simulink model "sevietta_devel_2017h"  (R2013a)
settings: Solver=VariableStepDiscrete  SolverMode=SingleTasking  StartTime=0.0  StopTime=3276  RelTol=1e-3
undefined symbols (not defined in the file): sfp
libraries: xbsIndex_r4 x2565, casper_library_delays x32, simulink x19, casper_library_misc x17, xps_library x13
(part 24 of 31)

== system sevietta_devel_2017h/pkt/packetizer/pkt_header ==
  note: CHIPS 2.0: Spare byte before first_chan
  note: trigger signal does selection on mux
  rst : Inport
  new_seq : Inport  Port=2
  new_pkt : Inport  Port=3
  roach_id : Inport  Port=4
  gbe_id : Inport  Port=5
  n_chan : Inport  Port=6
  n_subband : Inport  Port=7
  subband_id : Inport  Port=8
  first_chan : Inport  Port=9
  spare : Inport  Port=10
  Concat : xbsIndex_r4/Concat  num_inputs=7  dbl_ovrd=off  block_type=concat
  Delay1 : xbsIndex_r4/Delay  rst=off  infoeditControl=Selection of Reset will increase slice count due to use of real FFs and instead of SRLs  en=off  latency=4  dbl_ovrd=off  reg_retiming=off  block_type=delay
  Delay2 : xbsIndex_r4/Delay  rst=off  infoeditControl=Selection of Reset will increase slice count due to use of real FFs and instead of SRLs  en=off  latency=2  dbl_ovrd=off  reg_retiming=off  block_type=delay
  Delay3 : xbsIndex_r4/Delay  rst=off  infoeditControl=Selection of Reset will increase slice count due to use of real FFs and instead of SRLs  en=off  latency=4  dbl_ovrd=off  reg_retiming=off  block_type=delay
  Gateway Out{1..4,8} (5 alike) : xbsIndex_r4/Gateway Out  inherit_from_input=off  hdl_port=on  timing_constraint=None  locs_specified=off  LOCs={}  UseAsDAC=off  DACChannel='1'  block_type=gatewayout
  Mux : xbsIndex_r4/Mux  inputs=2  en=off  latency=1  precision=Full  arith_type=Unsigned  n_bits=16  bin_pt=14  quantization=Truncate  overflow=Wrap  dbl_ovrd=off  block_type=mux
  Scope2 : Scope  NumInputPorts=5
      settings: ShowLegends=on  TimeRange=50000  YMin=-5~0~-5~0~-5  YMax=5~8e+16~5~10~5  SaveName=ScopeData2  MaxDataPoints=10000
  Slice{,1..4,6} (6 alike) : xbsIndex_r4/Slice  nbits=8  boolean_output=off  mode=Lower Bit Location + Width  bit1=0  base1=MSB of Input  bit0=0  base0=LSB of Input  dbl_ovrd=off  block_type=slice
  Slice5 : xbsIndex_r4/Slice  nbits=16  boolean_output=off  mode=Lower Bit Location + Width  bit1=0  base1=MSB of Input  bit0=0  base0=LSB of Input  dbl_ovrd=off  block_type=slice
  pulse_ext : casper_library_misc/pulse_ext  pulse_len=2
  seq_no : xbsIndex_r4/Counter  cnt_type=Free Running  cnt_to=Inf  operation=Up  start_count=0  cnt_by_val=1  arith_type=Unsigned  n_bits=64  bin_pt=0  load_pin=off  rst=on  en=on  explicit_period=on  period=1  dbl_ovrd=off  use_behavioral_HDL=off  implementation=Fabric  block_type=counter
  hdr_valid : Outport
  hdr_out : Outport  Port=2
  wires:
  Delay2/1 -> pulse_ext/1, Gateway Out1/1, Mux/1
  first_chan/1 -> Slice5/1
  subband_id/1 -> Slice4/1
  spare/1 -> Slice6/1
  Slice4/1 -> Concat/5
  pulse_ext/1 -> Delay1/1
  Mux/1 -> Delay3/1
  gbe_id/1 -> Slice1/1
  new_seq/1 -> seq_no/2
  n_subband/1 -> Slice3/1
  Slice1/1 -> Concat/2
  Slice/1 -> Concat/1
  n_chan/1 -> Slice2/1
  rst/1 -> seq_no/1
  Slice2/1 -> Concat/3
  Slice3/1 -> Concat/4
  seq_no/1 -> Gateway Out2/1, Mux/2
  roach_id/1 -> Slice/1
  new_pkt/1 -> Delay2/1
  Delay1/1 -> Gateway Out4/1, hdr_valid/1
  Delay3/1 -> Gateway Out8/1, hdr_out/1
  Slice6/1 -> Concat/6
  Slice5/1 -> Concat/7
  Gateway Out1/1 -> Scope2/1  "new_pkt"
  Gateway Out2/1 -> Scope2/2  "seq_no"
  Gateway Out3/1 -> Scope2/3  "hdr_data"
  Gateway Out8/1 -> Scope2/4  "output"
  Gateway Out4/1 -> Scope2/5
  Concat/1 -> Mux/3, Gateway Out3/1

== system sevietta_devel_2017h/pkt/packetizer/re_logic ==
  sow : Inport
  n_chanps : Inport  Port=2
  n_subband : Inport  Port=3
  cnt_rst : Inport  Port=4
  start_chan : Inport  Port=5
  Delay4 : xbsIndex_r4/Delay  rst=off  infoeditControl=Selection of Reset will increase slice count due to use of real FFs and instead of SRLs  en=off  latency=5  dbl_ovrd=off  reg_retiming=off  block_type=delay
  Delay5 : xbsIndex_r4/Delay  rst=off  infoeditControl=Selection of Reset will increase slice count due to use of real FFs and instead of SRLs  en=off  latency=5  dbl_ovrd=off  reg_retiming=off  block_type=delay
  Delay6 : xbsIndex_r4/Delay  rst=off  infoeditControl=Selection of Reset will increase slice count due to use of real FFs and instead of SRLs  en=off  latency=5  dbl_ovrd=off  reg_retiming=off  block_type=delay
  Delay7 : xbsIndex_r4/Delay  rst=off  infoeditControl=Selection of Reset will increase slice count due to use of real FFs and instead of SRLs  en=off  latency=1  dbl_ovrd=off  reg_retiming=off  block_type=delay
  compute_pkt_chan1 : Subsystem
  gen_eof1 : Subsystem
  re_logic1 : Subsystem
  new_cycle_out : Outport
  sub_id_out : Outport  Port=2
  sub_re : Outport  Port=3
  sof : Outport  Port=4
  eof : Outport  Port=5
  pkt_chan0 : Outport  Port=6
  wires:
  Delay6/1 -> gen_eof1/3(subband_re)
  compute_pkt_chan1/1(pkt_chan0) -> Delay7/1
  Delay7/1 -> pkt_chan0/1
  sow/1 -> re_logic1/1(sow)
  gen_eof1/5(eof) -> eof/1
  gen_eof1/4(sof) -> sof/1
  gen_eof1/2(subband_id_out) -> sub_id_out/1
  gen_eof1/3(pkt_re) -> sub_re/1
  n_subband/1 -> re_logic1/3(n_subband)
  n_chanps/1 -> compute_pkt_chan1/1(n_chanps), re_logic1/2(n_chanps)
  cnt_rst/1 -> re_logic1/4(rst)
  start_chan/1 -> compute_pkt_chan1/3(start_chan)
  Delay4/1 -> gen_eof1/1(new_cycle)
  Delay5/1 -> gen_eof1/2(subband_id)
  re_logic1/1(new_cycle) -> Delay4/1
  re_logic1/3(subband_re) -> Delay6/1
  re_logic1/2(subband_id) -> compute_pkt_chan1/2(subband_id), Delay5/1
  gen_eof1/1(new_cycle_out) -> new_cycle_out/1

== system sevietta_devel_2017h/pkt/packetizer1/pkt_buffer ==
  note: LATENCY TO MATCH FIFO LATENCY
  re : Inport
  d_in : Inport  Port=2
  we : Inport  Port=3
  new_fft_win : Inport  Port=4
  Constant1 : xbsIndex_r4/Constant  const=0  gui_display_data_type=Fixed-point  arith_type=Unsigned  n_bits=64  bin_pt=0  preci_type=Single  exp_width=8  frac_width=24  explicit_period=on  period=1  equ=P=C  opselect=C  inp2=PCIN>>17  opr=+  inp1=P  carry=CIN  dbl_ovrd=off  block_type=constant
  Constant2 : xbsIndex_r4/Constant  const=0  gui_display_data_type=Boolean  arith_type=Boolean  n_bits=64  bin_pt=0  preci_type=Single  exp_width=8  frac_width=24  explicit_period=on  period=1  equ=P=C  opselect=C  inp2=PCIN>>17  opr=+  inp1=P  carry=CIN  dbl_ovrd=off  block_type=constant
  Delay1 : xbsIndex_r4/Delay  rst=off  infoeditControl=Selection of Reset will increase slice count due to use of real FFs and instead of SRLs  en=off  latency=5  dbl_ovrd=off  reg_retiming=off  block_type=delay
  Delay2 : xbsIndex_r4/Delay  rst=off  infoeditControl=Selection of Reset will increase slice count due to use of real FFs and instead of SRLs  en=off  latency=5  dbl_ovrd=off  reg_retiming=off  block_type=delay
  Delay5 : xbsIndex_r4/Delay  rst=off  infoeditControl=Selection of Reset will increase slice count due to use of real FFs and instead of SRLs  en=off  latency=3  dbl_ovrd=off  reg_retiming=off  block_type=delay
  Gateway Out{1..5,7..9,18..20} (11 alike) : xbsIndex_r4/Gateway Out  inherit_from_input=off  hdl_port=on  timing_constraint=None  locs_specified=off  LOCs={}  UseAsDAC=off  DACChannel='1'  block_type=gatewayout
  Scope1 : Scope  NumInputPorts=2
      settings: ShowLegends=on  YMin=-0.1~-0.1  YMax=1.1~1.1  MaxDataPoints=10000
  Scope3 : Scope  NumInputPorts=3
      settings: ShowLegends=on  YMin=-0.1~-0.1~-0.1  YMax=1.1~1.1~1.1  SaveName=ScopeData3  MaxDataPoints=10000
  Scope5 : Scope  NumInputPorts=6
      settings: ShowLegends=on  YMin=-5~-5~-0.1~-5~-5~-0.1  YMax=5~5~1.1~5~5~1.1  MaxDataPoints=10000
  dual_prt_ram : xbsIndex_r4/Dual Port RAM  depth=4096  initVector=sin(pi*(0:15)/16)  distributed_mem=Block RAM  init_a=0  init_b=0  rst_a=off  rst_b=off  en_a=off  en_b=off  latency=3  write_mode_A=Read After Write  write_mode_B=Read After Write  dbl_ovrd=off  optimize=Area  block_type=dpram
  re_addr : xbsIndex_r4/Counter  cnt_type=Free Running  cnt_to=Inf  operation=Up  start_count=0  cnt_by_val=1  arith_type=Unsigned  n_bits=12  bin_pt=0  load_pin=off  rst=on  en=on  explicit_period=on  period=1  dbl_ovrd=off  use_behavioral_HDL=off  implementation=Fabric  block_type=counter
  wr_addr : xbsIndex_r4/Counter  cnt_type=Free Running  cnt_to=Inf  operation=Up  start_count=0  cnt_by_val=1  arith_type=Unsigned  n_bits=10  bin_pt=0  load_pin=off  rst=on  en=on  explicit_period=on  period=1  dbl_ovrd=off  use_behavioral_HDL=off  implementation=Fabric  block_type=counter
  d_valid : Outport
  d_out : Outport  Port=2
  wires:
  Delay2/1 -> d_out/1, Gateway Out5/1
  Delay1/1 -> d_valid/1, Gateway Out4/1
  Constant2/1 -> dual_prt_ram/3, Gateway Out19/1
  re/1 -> Gateway Out9/1, re_addr/2, Delay5/1
  Gateway Out5/1 -> Scope1/2
  Gateway Out4/1 -> Scope1/1
  dual_prt_ram/1 -> Delay2/1
  d_in/1 -> Gateway Out1/1, dual_prt_ram/5
  Constant1/1 -> dual_prt_ram/2, Gateway Out18/1
  Gateway Out3/1 -> Scope5/4  "addr_b"
  Gateway Out1/1 -> Scope5/5  "data_b"
  Gateway Out2/1 -> Scope5/6  "we_b"
  [wr_en] -> dual_prt_ram/6, Gateway Out2/1
  [wr_addr] -> dual_prt_ram/4, Gateway Out3/1
  [re_addr] -> dual_prt_ram/1, Gateway Out20/1
  Gateway Out8/1 -> Scope3/3  "fftwin"
  Gateway Out7/1 -> Scope3/2  "ween"
  Gateway Out9/1 -> Scope3/1  "reen"
  [new_fft_win] -> re_addr/1
  [new_fft_win] -> wr_addr/1
  Gateway Out19/1 -> Scope5/3  "we_a"
  Gateway Out18/1 -> Scope5/2  "data_a"
  Gateway Out20/1 -> Scope5/1  "addr_a"
  wr_addr/1 -> [wr_addr]
  re_addr/1 -> [re_addr]
  new_fft_win/1 -> Gateway Out8/1, [new_fft_win]
  we/1 -> Gateway Out7/1, wr_addr/2, [wr_en]
  Delay5/1 -> Delay1/1

== system sevietta_devel_2017h/pkt/packetizer1/pkt_header ==
  note: trigger signal does selection on mux
  note: CHIPS 2.0: Spare byte before first_chan
  rst : Inport
  new_seq : Inport  Port=2
  new_pkt : Inport  Port=3
  roach_id : Inport  Port=4
  gbe_id : Inport  Port=5
  n_chan : Inport  Port=6
  n_subband : Inport  Port=7
  subband_id : Inport  Port=8
  first_chan : Inport  Port=9
  spare : Inport  Port=10
  Concat : xbsIndex_r4/Concat  num_inputs=7  dbl_ovrd=off  block_type=concat
  Delay1 : xbsIndex_r4/Delay  rst=off  infoeditControl=Selection of Reset will increase slice count due to use of real FFs and instead of SRLs  en=off  latency=4  dbl_ovrd=off  reg_retiming=off  block_type=delay
  Delay2 : xbsIndex_r4/Delay  rst=off  infoeditControl=Selection of Reset will increase slice count due to use of real FFs and instead of SRLs  en=off  latency=2  dbl_ovrd=off  reg_retiming=off  block_type=delay
  Delay3 : xbsIndex_r4/Delay  rst=off  infoeditControl=Selection of Reset will increase slice count due to use of real FFs and instead of SRLs  en=off  latency=4  dbl_ovrd=off  reg_retiming=off  block_type=delay
  Gateway Out{1..4,8} (5 alike) : xbsIndex_r4/Gateway Out  inherit_from_input=off  hdl_port=on  timing_constraint=None  locs_specified=off  LOCs={}  UseAsDAC=off  DACChannel='1'  block_type=gatewayout
  Mux : xbsIndex_r4/Mux  inputs=2  en=off  latency=1  precision=Full  arith_type=Unsigned  n_bits=16  bin_pt=14  quantization=Truncate  overflow=Wrap  dbl_ovrd=off  block_type=mux
  Scope2 : Scope  NumInputPorts=5
      settings: ShowLegends=on  TimeRange=50000  YMin=-5~0~-5~0~-5  YMax=5~8e+16~5~10~5  SaveName=ScopeData2  MaxDataPoints=10000
  Slice{,1..4,6} (6 alike) : xbsIndex_r4/Slice  nbits=8  boolean_output=off  mode=Lower Bit Location + Width  bit1=0  base1=MSB of Input  bit0=0  base0=LSB of Input  dbl_ovrd=off  block_type=slice
  Slice5 : xbsIndex_r4/Slice  nbits=16  boolean_output=off  mode=Lower Bit Location + Width  bit1=0  base1=MSB of Input  bit0=0  base0=LSB of Input  dbl_ovrd=off  block_type=slice
  pulse_ext : casper_library_misc/pulse_ext  pulse_len=2
  seq_no : xbsIndex_r4/Counter  cnt_type=Free Running  cnt_to=Inf  operation=Up  start_count=0  cnt_by_val=1  arith_type=Unsigned  n_bits=64  bin_pt=0  load_pin=off  rst=on  en=on  explicit_period=on  period=1  dbl_ovrd=off  use_behavioral_HDL=off  implementation=Fabric  block_type=counter
  hdr_valid : Outport
  hdr_out : Outport  Port=2
  wires:
  Concat/1 -> Gateway Out3/1, Mux/3
  Gateway Out4/1 -> Scope2/5
  Gateway Out8/1 -> Scope2/4  "output"
  Gateway Out3/1 -> Scope2/3  "hdr_data"
  Gateway Out2/1 -> Scope2/2  "seq_no"
  Gateway Out1/1 -> Scope2/1  "new_pkt"
  Slice5/1 -> Concat/7
  Slice6/1 -> Concat/6
  Delay3/1 -> hdr_out/1, Gateway Out8/1
  Delay1/1 -> hdr_valid/1, Gateway Out4/1
  new_pkt/1 -> Delay2/1
  roach_id/1 -> Slice/1
  seq_no/1 -> Mux/2, Gateway Out2/1
  Slice3/1 -> Concat/4
  Slice2/1 -> Concat/3
  rst/1 -> seq_no/1
  n_chan/1 -> Slice2/1
  Slice/1 -> Concat/1
  Slice1/1 -> Concat/2
  n_subband/1 -> Slice3/1
  new_seq/1 -> seq_no/2
  gbe_id/1 -> Slice1/1
  Mux/1 -> Delay3/1
  pulse_ext/1 -> Delay1/1
  Slice4/1 -> Concat/5
  spare/1 -> Slice6/1
  subband_id/1 -> Slice4/1
  first_chan/1 -> Slice5/1
  Delay2/1 -> Mux/1, Gateway Out1/1, pulse_ext/1

== system sevietta_devel_2017h/pkt/packetizer1/re_logic ==
  sow : Inport
  n_chanps : Inport  Port=2
  n_subband : Inport  Port=3
  cnt_rst : Inport  Port=4
  start_chan : Inport  Port=5
  Delay4 : xbsIndex_r4/Delay  rst=off  infoeditControl=Selection of Reset will increase slice count due to use of real FFs and instead of SRLs  en=off  latency=5  dbl_ovrd=off  reg_retiming=off  block_type=delay
  Delay5 : xbsIndex_r4/Delay  rst=off  infoeditControl=Selection of Reset will increase slice count due to use of real FFs and instead of SRLs  en=off  latency=5  dbl_ovrd=off  reg_retiming=off  block_type=delay
  Delay6 : xbsIndex_r4/Delay  rst=off  infoeditControl=Selection of Reset will increase slice count due to use of real FFs and instead of SRLs  en=off  latency=5  dbl_ovrd=off  reg_retiming=off  block_type=delay
  Delay7 : xbsIndex_r4/Delay  rst=off  infoeditControl=Selection of Reset will increase slice count due to use of real FFs and instead of SRLs  en=off  latency=1  dbl_ovrd=off  reg_retiming=off  block_type=delay
  compute_pkt_chan1 : Subsystem
  gen_eof1 : Subsystem
  re_logic1 : Subsystem
  new_cycle_out : Outport
  sub_id_out : Outport  Port=2
  sub_re : Outport  Port=3
  sof : Outport  Port=4
  eof : Outport  Port=5
  pkt_chan0 : Outport  Port=6
  wires:
  gen_eof1/1(new_cycle_out) -> new_cycle_out/1
  re_logic1/2(subband_id) -> Delay5/1, compute_pkt_chan1/2(subband_id)
  re_logic1/3(subband_re) -> Delay6/1
  re_logic1/1(new_cycle) -> Delay4/1
  Delay5/1 -> gen_eof1/2(subband_id)
  Delay4/1 -> gen_eof1/1(new_cycle)
  start_chan/1 -> compute_pkt_chan1/3(start_chan)
  cnt_rst/1 -> re_logic1/4(rst)
  n_chanps/1 -> re_logic1/2(n_chanps), compute_pkt_chan1/1(n_chanps)
  n_subband/1 -> re_logic1/3(n_subband)
  gen_eof1/3(pkt_re) -> sub_re/1
  gen_eof1/2(subband_id_out) -> sub_id_out/1
  gen_eof1/4(sof) -> sof/1
  gen_eof1/5(eof) -> eof/1
  sow/1 -> re_logic1/1(sow)
  Delay7/1 -> pkt_chan0/1
  compute_pkt_chan1/1(pkt_chan0) -> Delay7/1
  Delay6/1 -> gen_eof1/3(subband_re)

== system sevietta_devel_2017h/pkt/packetizer2/pkt_buffer ==
  note: LATENCY TO MATCH FIFO LATENCY
  re : Inport
  d_in : Inport  Port=2
  we : Inport  Port=3
  new_fft_win : Inport  Port=4
  Constant1 : xbsIndex_r4/Constant  const=0  gui_display_data_type=Fixed-point  arith_type=Unsigned  n_bits=64  bin_pt=0  preci_type=Single  exp_width=8  frac_width=24  explicit_period=on  period=1  equ=P=C  opselect=C  inp2=PCIN>>17  opr=+  inp1=P  carry=CIN  dbl_ovrd=off  block_type=constant
  Constant2 : xbsIndex_r4/Constant  const=0  gui_display_data_type=Boolean  arith_type=Boolean  n_bits=64  bin_pt=0  preci_type=Single  exp_width=8  frac_width=24  explicit_period=on  period=1  equ=P=C  opselect=C  inp2=PCIN>>17  opr=+  inp1=P  carry=CIN  dbl_ovrd=off  block_type=constant
  Delay1 : xbsIndex_r4/Delay  rst=off  infoeditControl=Selection of Reset will increase slice count due to use of real FFs and instead of SRLs  en=off  latency=5  dbl_ovrd=off  reg_retiming=off  block_type=delay
  Delay2 : xbsIndex_r4/Delay  rst=off  infoeditControl=Selection of Reset will increase slice count due to use of real FFs and instead of SRLs  en=off  latency=5  dbl_ovrd=off  reg_retiming=off  block_type=delay
  Delay5 : xbsIndex_r4/Delay  rst=off  infoeditControl=Selection of Reset will increase slice count due to use of real FFs and instead of SRLs  en=off  latency=3  dbl_ovrd=off  reg_retiming=off  block_type=delay
  Gateway Out{1..5,7..9,18..20} (11 alike) : xbsIndex_r4/Gateway Out  inherit_from_input=off  hdl_port=on  timing_constraint=None  locs_specified=off  LOCs={}  UseAsDAC=off  DACChannel='1'  block_type=gatewayout
  Scope1 : Scope  NumInputPorts=2
      settings: ShowLegends=on  YMin=-0.1~-0.1  YMax=1.1~1.1  MaxDataPoints=10000
  Scope3 : Scope  NumInputPorts=3
      settings: ShowLegends=on  YMin=-0.1~-0.1~-0.1  YMax=1.1~1.1~1.1  SaveName=ScopeData3  MaxDataPoints=10000
  Scope5 : Scope  NumInputPorts=6
      settings: ShowLegends=on  YMin=-5~-5~-0.1~-5~-5~-0.1  YMax=5~5~1.1~5~5~1.1  MaxDataPoints=10000
  dual_prt_ram : xbsIndex_r4/Dual Port RAM  depth=4096  initVector=sin(pi*(0:15)/16)  distributed_mem=Block RAM  init_a=0  init_b=0  rst_a=off  rst_b=off  en_a=off  en_b=off  latency=3  write_mode_A=Read After Write  write_mode_B=Read After Write  dbl_ovrd=off  optimize=Area  block_type=dpram
  re_addr : xbsIndex_r4/Counter  cnt_type=Free Running  cnt_to=Inf  operation=Up  start_count=0  cnt_by_val=1  arith_type=Unsigned  n_bits=12  bin_pt=0  load_pin=off  rst=on  en=on  explicit_period=on  period=1  dbl_ovrd=off  use_behavioral_HDL=off  implementation=Fabric  block_type=counter
  wr_addr : xbsIndex_r4/Counter  cnt_type=Free Running  cnt_to=Inf  operation=Up  start_count=0  cnt_by_val=1  arith_type=Unsigned  n_bits=10  bin_pt=0  load_pin=off  rst=on  en=on  explicit_period=on  period=1  dbl_ovrd=off  use_behavioral_HDL=off  implementation=Fabric  block_type=counter
  d_valid : Outport
  d_out : Outport  Port=2
  wires:
  Delay5/1 -> Delay1/1
  we/1 -> [wr_en], wr_addr/2, Gateway Out7/1
  new_fft_win/1 -> [new_fft_win], Gateway Out8/1
  re_addr/1 -> [re_addr]
  wr_addr/1 -> [wr_addr]
  Gateway Out20/1 -> Scope5/1  "addr_a"
  Gateway Out18/1 -> Scope5/2  "data_a"
  Gateway Out19/1 -> Scope5/3  "we_a"
  [new_fft_win] -> wr_addr/1
  [new_fft_win] -> re_addr/1
  Gateway Out9/1 -> Scope3/1  "reen"
  Gateway Out7/1 -> Scope3/2  "ween"
  Gateway Out8/1 -> Scope3/3  "fftwin"
  [re_addr] -> Gateway Out20/1, dual_prt_ram/1
  [wr_addr] -> Gateway Out3/1, dual_prt_ram/4
  [wr_en] -> Gateway Out2/1, dual_prt_ram/6
  Gateway Out2/1 -> Scope5/6  "we_b"
  Gateway Out1/1 -> Scope5/5  "data_b"
  Gateway Out3/1 -> Scope5/4  "addr_b"
  Constant1/1 -> Gateway Out18/1, dual_prt_ram/2
  d_in/1 -> dual_prt_ram/5, Gateway Out1/1
  dual_prt_ram/1 -> Delay2/1
  Gateway Out4/1 -> Scope1/1
  Gateway Out5/1 -> Scope1/2
  re/1 -> Delay5/1, re_addr/2, Gateway Out9/1
  Constant2/1 -> Gateway Out19/1, dual_prt_ram/3
  Delay1/1 -> Gateway Out4/1, d_valid/1
  Delay2/1 -> Gateway Out5/1, d_out/1

== system sevietta_devel_2017h/pkt/packetizer2/pkt_header ==
  note: CHIPS 2.0: Spare byte before first_chan
  note: trigger signal does selection on mux
  rst : Inport
  new_seq : Inport  Port=2
  new_pkt : Inport  Port=3
  roach_id : Inport  Port=4
  gbe_id : Inport  Port=5
  n_chan : Inport  Port=6
  n_subband : Inport  Port=7
  subband_id : Inport  Port=8
  first_chan : Inport  Port=9
  spare : Inport  Port=10
  Concat : xbsIndex_r4/Concat  num_inputs=7  dbl_ovrd=off  block_type=concat
  Delay1 : xbsIndex_r4/Delay  rst=off  infoeditControl=Selection of Reset will increase slice count due to use of real FFs and instead of SRLs  en=off  latency=4  dbl_ovrd=off  reg_retiming=off  block_type=delay
  Delay2 : xbsIndex_r4/Delay  rst=off  infoeditControl=Selection of Reset will increase slice count due to use of real FFs and instead of SRLs  en=off  latency=2  dbl_ovrd=off  reg_retiming=off  block_type=delay
  Delay3 : xbsIndex_r4/Delay  rst=off  infoeditControl=Selection of Reset will increase slice count due to use of real FFs and instead of SRLs  en=off  latency=4  dbl_ovrd=off  reg_retiming=off  block_type=delay
  Gateway Out{1..4,8} (5 alike) : xbsIndex_r4/Gateway Out  inherit_from_input=off  hdl_port=on  timing_constraint=None  locs_specified=off  LOCs={}  UseAsDAC=off  DACChannel='1'  block_type=gatewayout
  Mux : xbsIndex_r4/Mux  inputs=2  en=off  latency=1  precision=Full  arith_type=Unsigned  n_bits=16  bin_pt=14  quantization=Truncate  overflow=Wrap  dbl_ovrd=off  block_type=mux
  Scope2 : Scope  NumInputPorts=5
      settings: ShowLegends=on  TimeRange=50000  YMin=-5~0~-5~0~-5  YMax=5~8e+16~5~10~5  SaveName=ScopeData2  MaxDataPoints=10000
  Slice{,1..4,6} (6 alike) : xbsIndex_r4/Slice  nbits=8  boolean_output=off  mode=Lower Bit Location + Width  bit1=0  base1=MSB of Input  bit0=0  base0=LSB of Input  dbl_ovrd=off  block_type=slice
  Slice5 : xbsIndex_r4/Slice  nbits=16  boolean_output=off  mode=Lower Bit Location + Width  bit1=0  base1=MSB of Input  bit0=0  base0=LSB of Input  dbl_ovrd=off  block_type=slice
  pulse_ext : casper_library_misc/pulse_ext  pulse_len=2
  seq_no : xbsIndex_r4/Counter  cnt_type=Free Running  cnt_to=Inf  operation=Up  start_count=0  cnt_by_val=1  arith_type=Unsigned  n_bits=64  bin_pt=0  load_pin=off  rst=on  en=on  explicit_period=on  period=1  dbl_ovrd=off  use_behavioral_HDL=off  implementation=Fabric  block_type=counter
  hdr_valid : Outport
  hdr_out : Outport  Port=2
  wires:
  Delay2/1 -> pulse_ext/1, Gateway Out1/1, Mux/1
  first_chan/1 -> Slice5/1
  subband_id/1 -> Slice4/1
  spare/1 -> Slice6/1
  Slice4/1 -> Concat/5
  pulse_ext/1 -> Delay1/1
  Mux/1 -> Delay3/1
  gbe_id/1 -> Slice1/1
  new_seq/1 -> seq_no/2
  n_subband/1 -> Slice3/1
  Slice1/1 -> Concat/2
  Slice/1 -> Concat/1
  n_chan/1 -> Slice2/1
  rst/1 -> seq_no/1
  Slice2/1 -> Concat/3
  Slice3/1 -> Concat/4
  seq_no/1 -> Gateway Out2/1, Mux/2
  roach_id/1 -> Slice/1
  new_pkt/1 -> Delay2/1
  Delay1/1 -> Gateway Out4/1, hdr_valid/1
  Delay3/1 -> Gateway Out8/1, hdr_out/1
  Slice6/1 -> Concat/6
  Slice5/1 -> Concat/7
  Gateway Out1/1 -> Scope2/1  "new_pkt"
  Gateway Out2/1 -> Scope2/2  "seq_no"
  Gateway Out3/1 -> Scope2/3  "hdr_data"
  Gateway Out8/1 -> Scope2/4  "output"
  Gateway Out4/1 -> Scope2/5
  Concat/1 -> Mux/3, Gateway Out3/1

== system sevietta_devel_2017h/pkt/packetizer2/re_logic ==
  sow : Inport
  n_chanps : Inport  Port=2
  n_subband : Inport  Port=3
  cnt_rst : Inport  Port=4
  start_chan : Inport  Port=5
  Delay4 : xbsIndex_r4/Delay  rst=off  infoeditControl=Selection of Reset will increase slice count due to use of real FFs and instead of SRLs  en=off  latency=5  dbl_ovrd=off  reg_retiming=off  block_type=delay
  Delay5 : xbsIndex_r4/Delay  rst=off  infoeditControl=Selection of Reset will increase slice count due to use of real FFs and instead of SRLs  en=off  latency=5  dbl_ovrd=off  reg_retiming=off  block_type=delay
  Delay6 : xbsIndex_r4/Delay  rst=off  infoeditControl=Selection of Reset will increase slice count due to use of real FFs and instead of SRLs  en=off  latency=5  dbl_ovrd=off  reg_retiming=off  block_type=delay
  Delay7 : xbsIndex_r4/Delay  rst=off  infoeditControl=Selection of Reset will increase slice count due to use of real FFs and instead of SRLs  en=off  latency=1  dbl_ovrd=off  reg_retiming=off  block_type=delay
  compute_pkt_chan1 : Subsystem
  gen_eof1 : Subsystem
  re_logic1 : Subsystem
  new_cycle_out : Outport
  sub_id_out : Outport  Port=2
  sub_re : Outport  Port=3
  sof : Outport  Port=4
  eof : Outport  Port=5
  pkt_chan0 : Outport  Port=6
  wires:
  Delay6/1 -> gen_eof1/3(subband_re)
  compute_pkt_chan1/1(pkt_chan0) -> Delay7/1
  Delay7/1 -> pkt_chan0/1
  sow/1 -> re_logic1/1(sow)
  gen_eof1/5(eof) -> eof/1
  gen_eof1/4(sof) -> sof/1
  gen_eof1/2(subband_id_out) -> sub_id_out/1
  gen_eof1/3(pkt_re) -> sub_re/1
  n_subband/1 -> re_logic1/3(n_subband)
  n_chanps/1 -> compute_pkt_chan1/1(n_chanps), re_logic1/2(n_chanps)
  cnt_rst/1 -> re_logic1/4(rst)
  start_chan/1 -> compute_pkt_chan1/3(start_chan)
  Delay4/1 -> gen_eof1/1(new_cycle)
  Delay5/1 -> gen_eof1/2(subband_id)
  re_logic1/1(new_cycle) -> Delay4/1
  re_logic1/3(subband_re) -> Delay6/1
  re_logic1/2(subband_id) -> compute_pkt_chan1/2(subband_id), Delay5/1
  gen_eof1/1(new_cycle_out) -> new_cycle_out/1

== system sevietta_devel_2017h/pkt/packetizer3/pkt_buffer ==
  note: LATENCY TO MATCH FIFO LATENCY
  re : Inport
  d_in : Inport  Port=2
  we : Inport  Port=3
  new_fft_win : Inport  Port=4
  Constant1 : xbsIndex_r4/Constant  const=0  gui_display_data_type=Fixed-point  arith_type=Unsigned  n_bits=64  bin_pt=0  preci_type=Single  exp_width=8  frac_width=24  explicit_period=on  period=1  equ=P=C  opselect=C  inp2=PCIN>>17  opr=+  inp1=P  carry=CIN  dbl_ovrd=off  block_type=constant
  Constant2 : xbsIndex_r4/Constant  const=0  gui_display_data_type=Boolean  arith_type=Boolean  n_bits=64  bin_pt=0  preci_type=Single  exp_width=8  frac_width=24  explicit_period=on  period=1  equ=P=C  opselect=C  inp2=PCIN>>17  opr=+  inp1=P  carry=CIN  dbl_ovrd=off  block_type=constant
  Delay1 : xbsIndex_r4/Delay  rst=off  infoeditControl=Selection of Reset will increase slice count due to use of real FFs and instead of SRLs  en=off  latency=5  dbl_ovrd=off  reg_retiming=off  block_type=delay
  Delay2 : xbsIndex_r4/Delay  rst=off  infoeditControl=Selection of Reset will increase slice count due to use of real FFs and instead of SRLs  en=off  latency=5  dbl_ovrd=off  reg_retiming=off  block_type=delay
  Delay5 : xbsIndex_r4/Delay  rst=off  infoeditControl=Selection of Reset will increase slice count due to use of real FFs and instead of SRLs  en=off  latency=3  dbl_ovrd=off  reg_retiming=off  block_type=delay
  Gateway Out{1..5,7..9,18..20} (11 alike) : xbsIndex_r4/Gateway Out  inherit_from_input=off  hdl_port=on  timing_constraint=None  locs_specified=off  LOCs={}  UseAsDAC=off  DACChannel='1'  block_type=gatewayout
  Scope1 : Scope  NumInputPorts=2
      settings: ShowLegends=on  YMin=-0.1~-0.1  YMax=1.1~1.1  MaxDataPoints=10000
  Scope3 : Scope  NumInputPorts=3
      settings: ShowLegends=on  YMin=-0.1~-0.1~-0.1  YMax=1.1~1.1~1.1  SaveName=ScopeData3  MaxDataPoints=10000
  Scope5 : Scope  NumInputPorts=6
      settings: ShowLegends=on  YMin=-5~-5~-0.1~-5~-5~-0.1  YMax=5~5~1.1~5~5~1.1  MaxDataPoints=10000
  dual_prt_ram : xbsIndex_r4/Dual Port RAM  depth=4096  initVector=sin(pi*(0:15)/16)  distributed_mem=Block RAM  init_a=0  init_b=0  rst_a=off  rst_b=off  en_a=off  en_b=off  latency=3  write_mode_A=Read After Write  write_mode_B=Read After Write  dbl_ovrd=off  optimize=Area  block_type=dpram
  re_addr : xbsIndex_r4/Counter  cnt_type=Free Running  cnt_to=Inf  operation=Up  start_count=0  cnt_by_val=1  arith_type=Unsigned  n_bits=12  bin_pt=0  load_pin=off  rst=on  en=on  explicit_period=on  period=1  dbl_ovrd=off  use_behavioral_HDL=off  implementation=Fabric  block_type=counter
  wr_addr : xbsIndex_r4/Counter  cnt_type=Free Running  cnt_to=Inf  operation=Up  start_count=0  cnt_by_val=1  arith_type=Unsigned  n_bits=10  bin_pt=0  load_pin=off  rst=on  en=on  explicit_period=on  period=1  dbl_ovrd=off  use_behavioral_HDL=off  implementation=Fabric  block_type=counter
  d_valid : Outport
  d_out : Outport  Port=2
  wires:
  Delay2/1 -> d_out/1, Gateway Out5/1
  Delay1/1 -> d_valid/1, Gateway Out4/1
  Constant2/1 -> dual_prt_ram/3, Gateway Out19/1
  re/1 -> Gateway Out9/1, re_addr/2, Delay5/1
  Gateway Out5/1 -> Scope1/2
  Gateway Out4/1 -> Scope1/1
  dual_prt_ram/1 -> Delay2/1
  d_in/1 -> Gateway Out1/1, dual_prt_ram/5
  Constant1/1 -> dual_prt_ram/2, Gateway Out18/1
  Gateway Out3/1 -> Scope5/4  "addr_b"
  Gateway Out1/1 -> Scope5/5  "data_b"
  Gateway Out2/1 -> Scope5/6  "we_b"
  [wr_en] -> dual_prt_ram/6, Gateway Out2/1
  [wr_addr] -> dual_prt_ram/4, Gateway Out3/1
  [re_addr] -> dual_prt_ram/1, Gateway Out20/1
  Gateway Out8/1 -> Scope3/3  "fftwin"
  Gateway Out7/1 -> Scope3/2  "ween"
  Gateway Out9/1 -> Scope3/1  "reen"
  [new_fft_win] -> re_addr/1
  [new_fft_win] -> wr_addr/1
  Gateway Out19/1 -> Scope5/3  "we_a"
  Gateway Out18/1 -> Scope5/2  "data_a"
  Gateway Out20/1 -> Scope5/1  "addr_a"
  wr_addr/1 -> [wr_addr]
  re_addr/1 -> [re_addr]
  new_fft_win/1 -> Gateway Out8/1, [new_fft_win]
  we/1 -> Gateway Out7/1, wr_addr/2, [wr_en]
  Delay5/1 -> Delay1/1

== system sevietta_devel_2017h/pkt/packetizer3/pkt_header ==
  note: trigger signal does selection on mux
  note: CHIPS 2.0: Spare byte before first_chan
  rst : Inport
  new_seq : Inport  Port=2
  new_pkt : Inport  Port=3
  roach_id : Inport  Port=4
  gbe_id : Inport  Port=5
  n_chan : Inport  Port=6
  n_subband : Inport  Port=7
  subband_id : Inport  Port=8
  first_chan : Inport  Port=9
  spare : Inport  Port=10
  Concat : xbsIndex_r4/Concat  num_inputs=7  dbl_ovrd=off  block_type=concat
  Delay1 : xbsIndex_r4/Delay  rst=off  infoeditControl=Selection of Reset will increase slice count due to use of real FFs and instead of SRLs  en=off  latency=4  dbl_ovrd=off  reg_retiming=off  block_type=delay
  Delay2 : xbsIndex_r4/Delay  rst=off  infoeditControl=Selection of Reset will increase slice count due to use of real FFs and instead of SRLs  en=off  latency=2  dbl_ovrd=off  reg_retiming=off  block_type=delay
  Delay3 : xbsIndex_r4/Delay  rst=off  infoeditControl=Selection of Reset will increase slice count due to use of real FFs and instead of SRLs  en=off  latency=4  dbl_ovrd=off  reg_retiming=off  block_type=delay
  Gateway Out{1..4,8} (5 alike) : xbsIndex_r4/Gateway Out  inherit_from_input=off  hdl_port=on  timing_constraint=None  locs_specified=off  LOCs={}  UseAsDAC=off  DACChannel='1'  block_type=gatewayout
  Mux : xbsIndex_r4/Mux  inputs=2  en=off  latency=1  precision=Full  arith_type=Unsigned  n_bits=16  bin_pt=14  quantization=Truncate  overflow=Wrap  dbl_ovrd=off  block_type=mux
  Scope2 : Scope  NumInputPorts=5
      settings: ShowLegends=on  TimeRange=50000  YMin=-5~0~-5~0~-5  YMax=5~8e+16~5~10~5  SaveName=ScopeData2  MaxDataPoints=10000
  Slice{,1..4,6} (6 alike) : xbsIndex_r4/Slice  nbits=8  boolean_output=off  mode=Lower Bit Location + Width  bit1=0  base1=MSB of Input  bit0=0  base0=LSB of Input  dbl_ovrd=off  block_type=slice
  Slice5 : xbsIndex_r4/Slice  nbits=16  boolean_output=off  mode=Lower Bit Location + Width  bit1=0  base1=MSB of Input  bit0=0  base0=LSB of Input  dbl_ovrd=off  block_type=slice
  pulse_ext : casper_library_misc/pulse_ext  pulse_len=2
  seq_no : xbsIndex_r4/Counter  cnt_type=Free Running  cnt_to=Inf  operation=Up  start_count=0  cnt_by_val=1  arith_type=Unsigned  n_bits=64  bin_pt=0  load_pin=off  rst=on  en=on  explicit_period=on  period=1  dbl_ovrd=off  use_behavioral_HDL=off  implementation=Fabric  block_type=counter
  hdr_valid : Outport
  hdr_out : Outport  Port=2
  wires:
  Concat/1 -> Gateway Out3/1, Mux/3
  Gateway Out4/1 -> Scope2/5
  Gateway Out8/1 -> Scope2/4  "output"
  Gateway Out3/1 -> Scope2/3  "hdr_data"
  Gateway Out2/1 -> Scope2/2  "seq_no"
  Gateway Out1/1 -> Scope2/1  "new_pkt"
  Slice5/1 -> Concat/7
  Slice6/1 -> Concat/6
  Delay3/1 -> hdr_out/1, Gateway Out8/1
  Delay1/1 -> hdr_valid/1, Gateway Out4/1
  new_pkt/1 -> Delay2/1
  roach_id/1 -> Slice/1
  seq_no/1 -> Mux/2, Gateway Out2/1
  Slice3/1 -> Concat/4
  Slice2/1 -> Concat/3
  rst/1 -> seq_no/1
  n_chan/1 -> Slice2/1
  Slice/1 -> Concat/1
  Slice1/1 -> Concat/2
  n_subband/1 -> Slice3/1
  new_seq/1 -> seq_no/2
  gbe_id/1 -> Slice1/1
  Mux/1 -> Delay3/1
  pulse_ext/1 -> Delay1/1
  Slice4/1 -> Concat/5
  spare/1 -> Slice6/1
  subband_id/1 -> Slice4/1
  first_chan/1 -> Slice5/1
  Delay2/1 -> Mux/1, Gateway Out1/1, pulse_ext/1

== system sevietta_devel_2017h/pkt/packetizer3/re_logic ==
  sow : Inport
  n_chanps : Inport  Port=2
  n_subband : Inport  Port=3
  cnt_rst : Inport  Port=4
  start_chan : Inport  Port=5
  Delay4 : xbsIndex_r4/Delay  rst=off  infoeditControl=Selection of Reset will increase slice count due to use of real FFs and instead of SRLs  en=off  latency=5  dbl_ovrd=off  reg_retiming=off  block_type=delay
  Delay5 : xbsIndex_r4/Delay  rst=off  infoeditControl=Selection of Reset will increase slice count due to use of real FFs and instead of SRLs  en=off  latency=5  dbl_ovrd=off  reg_retiming=off  block_type=delay
  Delay6 : xbsIndex_r4/Delay  rst=off  infoeditControl=Selection of Reset will increase slice count due to use of real FFs and instead of SRLs  en=off  latency=5  dbl_ovrd=off  reg_retiming=off  block_type=delay
  Delay7 : xbsIndex_r4/Delay  rst=off  infoeditControl=Selection of Reset will increase slice count due to use of real FFs and instead of SRLs  en=off  latency=1  dbl_ovrd=off  reg_retiming=off  block_type=delay
  compute_pkt_chan1 : Subsystem
  gen_eof1 : Subsystem
  re_logic1 : Subsystem
  new_cycle_out : Outport
  sub_id_out : Outport  Port=2
  sub_re : Outport  Port=3
  sof : Outport  Port=4
  eof : Outport  Port=5
  pkt_chan0 : Outport  Port=6
  wires:
  gen_eof1/1(new_cycle_out) -> new_cycle_out/1
  re_logic1/2(subband_id) -> Delay5/1, compute_pkt_chan1/2(subband_id)
  re_logic1/3(subband_re) -> Delay6/1
  re_logic1/1(new_cycle) -> Delay4/1
  Delay5/1 -> gen_eof1/2(subband_id)
  Delay4/1 -> gen_eof1/1(new_cycle)
  start_chan/1 -> compute_pkt_chan1/3(start_chan)
  cnt_rst/1 -> re_logic1/4(rst)
  n_chanps/1 -> re_logic1/2(n_chanps), compute_pkt_chan1/1(n_chanps)
  n_subband/1 -> re_logic1/3(n_subband)
  gen_eof1/3(pkt_re) -> sub_re/1
  gen_eof1/2(subband_id_out) -> sub_id_out/1
  gen_eof1/4(sof) -> sof/1
  gen_eof1/5(eof) -> eof/1
  sow/1 -> re_logic1/1(sow)
  Delay7/1 -> pkt_chan0/1
  compute_pkt_chan1/1(pkt_chan0) -> Delay7/1
  Delay6/1 -> gen_eof1/3(subband_re)

== system sevietta_devel_2017h/fft/f1/cg/bpass ==
  rst : Inport
  Constant4 : xbsIndex_r4/Constant  const=0  gui_display_data_type=Fixed-point  arith_type=Unsigned  n_bits=16  bin_pt=0  preci_type=Single  exp_width=8  frac_width=24  explicit_period=on  period=1  equ=P=C  opselect=C  inp2=PCIN>>17  opr=+  inp1=P  carry=CIN  dbl_ovrd=off  block_type=constant
  Constant5 : xbsIndex_r4/Constant  const=0  gui_display_data_type=Fixed-point  arith_type=Boolean  n_bits=1  bin_pt=0  preci_type=Single  exp_width=8  frac_width=24  explicit_period=on  period=1  equ=P=C  opselect=C  inp2=PCIN>>17  opr=+  inp1=P  carry=CIN  dbl_ovrd=off  block_type=constant
  Counter2 : xbsIndex_r4/Counter  cnt_type=Free Running  cnt_to=Inf  operation=Up  start_count=0  cnt_by_val=1  arith_type=Unsigned  n_bits=12  bin_pt=0  load_pin=off  rst=on  en=off  explicit_period=off  period=1  dbl_ovrd=off  use_behavioral_HDL=off  implementation=Fabric  use_rpm=on  block_type=counter
      settings: xl_area=[0, 0, 0, 0, 0, 0, 0]
  bram : Subsystem  Tag=xps:bram  AncestorBlock=xps_library/Shared_BRAM  mask{arith_type=Unsigned, addr_width=12, data_width=32, reg_prim_output=off, reg_core_output=off, optimization=Minimum_Area, data_bin_pt=0, init_vals=[0:2^12-1], sample_rate=1}
      mask prompts: arith_type "Output Data Type"; addr_width "Address width"; data_width "Data Width"; reg_prim_output "Register Primitive Output"; reg_core_output "Register Core Output"; data_bin_pt "Data Binary Point"; init_vals "Initial values (simulation only)"; sample_rate "Sample rate"
      mask init:
      | shared_bram_mask;
      mask TypeOptions arith_type: Unsigned | Signed  (2's comp)
      mask TypeOptions data_width: 8 | 16 | 32 | 64 | 128
      mask TypeOptions optimization: Minimum_Area | Low_Power
  pipeline : Subsystem  AncestorBlock=casper_library_delays/pipeline  mask(pipeline){latency=1}
      mask help:
      | An explicitly laid-out delay line to avoid mapping to SRL16s
      | for use in pipelining to help achieve timing closure.
      mask init:
      | pipeline_init(gcb,'latency',latency);
      settings: AttributesFormatString=Latency = %<latency>
      mask Display:
      | port_label('input', 1, 'd');
      | port_label('output', 1, 'q');
      | disp(['Z^-', num2str(latency)]);
  pipeline1 : Subsystem  AncestorBlock=casper_library_delays/pipeline  mask(pipeline){latency=1}
      mask help:
      | An explicitly laid-out delay line to avoid mapping to SRL16s
      | for use in pipelining to help achieve timing closure.
      mask init:
      | pipeline_init(gcb,'latency',latency);
      settings: AttributesFormatString=Latency = %<latency>
      mask Display:
      | port_label('input', 1, 'd');
      | port_label('output', 1, 'q');
      | disp(['Z^-', num2str(latency)]);
  pipeline2 : Subsystem  AncestorBlock=casper_library_delays/pipeline  mask(pipeline){latency=1}
      mask help:
      | An explicitly laid-out delay line to avoid mapping to SRL16s
      | for use in pipelining to help achieve timing closure.
      mask init:
      | pipeline_init(gcb,'latency',latency);
      settings: AttributesFormatString=Latency = %<latency>
      mask Display:
      | port_label('input', 1, 'd');
      | port_label('output', 1, 'q');
      | disp(['Z^-', num2str(latency)]);
  pipeline3 : Subsystem  AncestorBlock=casper_library_delays/pipeline  mask(pipeline){latency=1}
      mask help:
      | An explicitly laid-out delay line to avoid mapping to SRL16s
      | for use in pipelining to help achieve timing closure.
      mask init:
      | pipeline_init(gcb,'latency',latency);
      settings: AttributesFormatString=Latency = %<latency>
      mask Display:
      | port_label('input', 1, 'd');
      | port_label('output', 1, 'q');
      | disp(['Z^-', num2str(latency)]);
  coeffs_out : Outport
  wires:
  pipeline3/1(q) -> bram/1(addr)
  pipeline2/1(q) -> bram/3(we)
  pipeline1/1(q) -> bram/2(data_in)
  pipeline/1(q) -> coeffs_out/1
  Counter2/1 -> pipeline3/1(d)
  bram/1(data_out) -> pipeline/1(d)
  rst/1 -> Counter2/1
  Constant5/1 -> pipeline2/1(d)
  Constant4/1 -> pipeline1/1(d)

== system sevietta_devel_2017h/fft/f1/rms_mon_4b/add_gen ==
  note: To storage
  note: prevent one extra
      | write to address 0
  note: Do one
      | capture by
      | default
  note: Count of bytes in BRAM
      | as well as done signal
  note: A total count of
      | bytes written to
      | BRAM since trig
  note: Force MSbit of count
      | to be '1' by negating busy
      | as counter bit may be '0' or '1'
  vin : Inport
  din : Inport  Port=2
  we : Inport  Port=3
  go : Inport  Port=4
  cont : Inport  Port=5
  init : Inport  Port=6
  Concat : xbsIndex_r4/Concat  num_inputs=3  dbl_ovrd=off  block_type=concat
      settings: block_version=10.1.3
  Convert : xbsIndex_r4/Convert  gui_display_data_type=Fixed-point  arith_type=Unsigned  n_bits=32-nsamples-log2(increment)-1  bin_pt=0  float_type=Single  exp_bits=8  fraction_bits=24  quantization=Truncate  overflow=Wrap  en=off  latency=0  dbl_ovrd=off  pipeline=off  block_type=convert
      settings: block_version=10.1.3
  Delay{,1..7} (8 alike) : xbsIndex_r4/Delay  rst=off  infoeditControl=Selection of Reset will increase slice count due to use of real FFs and instead of SRLs  en=off  latency=1  dbl_ovrd=off  reg_retiming=on  block_type=delay
      settings: block_version=11.4
  Inverter : xbsIndex_r4/Inverter  en=off  latency=1  dbl_ovrd=off  block_type=inv
      settings: block_version=11.4
  Inverter1 : xbsIndex_r4/Inverter  en=off  latency=0  dbl_ovrd=off  block_type=inv
      settings: block_version=11.4
  Logical1 : xbsIndex_r4/Logical  logical_function=AND  inputs=2  en=off  latency=1  precision=Full  arith_type=Unsigned  n_bits=8  bin_pt=2  align_bp=on  dbl_ovrd=off  block_type=logical
      settings: xl_area=[0, 0, 0, 0, 0, 0, 0]
  Logical2 : xbsIndex_r4/Logical  logical_function=AND  inputs=2  en=off  latency=1  precision=Full  arith_type=Unsigned  n_bits=8  bin_pt=2  align_bp=on  dbl_ovrd=off  block_type=logical
      settings: xl_area=[0, 0, 0, 0, 0, 0, 0]
  Logical4 : xbsIndex_r4/Logical  logical_function=OR  inputs=2  en=off  latency=0  precision=Full  arith_type=Unsigned  n_bits=8  bin_pt=2  align_bp=on  dbl_ovrd=off  block_type=logical
      settings: xl_area=[0, 0, 0, 0, 0, 0, 0]
  Logical6 : xbsIndex_r4/Logical  logical_function=AND  inputs=3  en=off  latency=0  precision=Full  arith_type=Unsigned  n_bits=8  bin_pt=2  align_bp=on  dbl_ovrd=off  block_type=logical
      settings: xl_area=[0, 0, 0, 0, 0, 0, 0]
  Register3 : xbsIndex_r4/Register  init=0  rst=on  en=on  dbl_ovrd=off  block_type=register
      settings: xl_area=[0, 0, 0, 0, 0, 0, 0]
  Register4 : xbsIndex_r4/Register  init=0  rst=off  en=on  dbl_ovrd=off  block_type=register
      settings: xl_area=[0, 0, 0, 0, 0, 0, 0]
  Register5 : xbsIndex_r4/Register  init=1  rst=on  en=on  dbl_ovrd=off  block_type=register
      settings: xl_area=[0, 0, 0, 0, 0, 0, 0]
  Shift : xbsIndex_r4/Shift  shift_dir=Left  shift_bits=32-nsamples-log2(increment)-1-1  en=off  latency=1  precision=Full  arith_type="Signed  (2's comp)"  n_bits=16  bin_pt=14  quantization=Truncate  overflow=Wrap  dbl_ovrd=off  block_type=shift
  add_gen : xbsIndex_r4/Counter  cnt_type=Free Running  cnt_to=1  operation=Up  start_count=0  cnt_by_val=increment  arith_type=Unsigned  n_bits=counter_size  bin_pt=0  load_pin=off  rst=on  en=on  explicit_period=on  period=1  dbl_ovrd=off  use_behavioral_HDL=off  implementation=Fabric  use_rpm=on  block_type=counter
      settings: xl_area=[0, 0, 0, 0, 0, 0, 0]
  edge_detect : Subsystem  AncestorBlock=casper_library_misc/edge_detect  mask(edge_detect){edge=Both, polarity=Active High, x_in=[0 0.08 0.08 0.16 0.16 0.24 0.24 0.32 0.32 0.4], y_in=[-1 -1  1  1  1  1 -1 -1 -1 -1], x_out=[0.6 0.68 0.68 0.76 0.76 0.84 0.84 0.92 0.92 1], y_out=[-1 -1  1  1 -1 -1  1  1 -1 -1]}
      mask prompts: edge "Edge Type"; polarity "Output Polarity"; x_in "Input X Positions"; y_in "Input Y Positions"; x_out "Output X Positions"; y_out "Output Y Positions"
      mask help: Output is active for one-cycle after each edge of the specified type (i.e. rising, falling or both).
      mask init: same as sevietta_devel_2017h/adc/edge_detect1
      settings: AttributesFormatString=|
      | both edges
      | active high
      mask Help: Output is active for one-cycle after each edge of the specified type (i.e. rising, falling, or both).  Latency is zero.
      mask TypeOptions edge: Rising | Falling | Both
      mask TypeOptions polarity: Active High | Active Low
      mask Display:
      | plot(x_in_num,0.5+y_in_num*0.2);
      | plot(x_out_num,0.5+y_out_num*0.2);
  slice1 : xbsIndex_r4/Slice  nbits=nsamples+log2(increment)  boolean_output=off  mode=Lower Bit Location + Width  bit1=0  base1=LSB of Input  bit0=0  base0=LSB of Input  dbl_ovrd=off  block_type=slice
      settings: block_version=10.1.3
  slice2 : xbsIndex_r4/Slice  nbits=nsamples-burst_size  boolean_output=off  mode=Lower Bit Location + Width  bit1=0  base1=LSB of Input  bit0=log2(increment)+burst_size  base0=LSB of Input  dbl_ovrd=off  block_type=slice
      settings: block_version=10.1.3
  slice3 : xbsIndex_r4/Slice  nbits=1  boolean_output=on  mode=Lower Bit Location + Width  bit1=0  base1=MSB of Input  bit0=nsamples + log2(increment)  base0=LSB of Input  dbl_ovrd=off  block_type=slice
      settings: block_version=10.1.3
  vout : Outport
  add : Outport  Port=2
  dout : Outport  Port=3
  we_o : Outport  Port=4
  status : Outport  Port=5
  en_cnt : Outport  Port=6
  wires:
  Shift/1 -> Concat/1
  Delay/1 -> Register5/2
  Inverter1/1 -> Logical4/2
  cont/1 -> Delay3/1
  edge_detect/1(out) -> Inverter1/1, Register5/3
  Register4/1 -> vout/1
  Logical2/1 -> Register4/2
  Register3/1 -> Logical2/2
  vin/1 -> Delay5/1
  add_gen/1 -> slice2/1, slice1/1, Delay2/1, slice3/1
  Register5/1 -> Convert/1, Inverter/1, Logical6/1
  slice3/1 -> edge_detect/1(in)
  init/1 -> Delay4/1
  Logical6/1 -> we_o/1, Logical2/1, Register3/2, add_gen/2
  Concat/1 -> status/1
  Convert/1 -> Shift/1
  slice2/1 -> add/1
  Delay2/1 -> en_cnt/1
  din/1 -> Delay6/1
  Delay1/1 -> Concat/3
  slice1/1 -> Delay1/1
  Inverter/1 -> Concat/2
  Logical4/1 -> Logical6/2
  we/1 -> Logical1/1
  go/1 -> Logical1/2
  Logical1/1 -> Logical6/3
  Delay7/1 -> Register4/1
  Delay3/1 -> Logical4/1, Register5/1
  Delay4/1 -> Register3/3, Register3/1, add_gen/1, Delay/1
  Delay5/1 -> Delay7/1
  Delay6/1 -> dout/1
